simulink model "lab07q1"  (Simulink 7.1)
settings: Solver=ode45  StartTime=0.0  StopTime=100  RelTol=1e-3
InitFcn:
  | RC = 2;
  | K= 1;
  | 
  | 
  | A = [(-1/RC)*(2-K) (1/RC)*K (-1/RC);(1/RC)*K (1/RC)*K (-1/RC);(1/(2*RC))*(1+2*K) (1/(2*RC))*(1+2*K) (-1/RC)]
  | 
  | B = [(1/RC)*(2-K);(-1/RC)*K;(-1/RC)*K]
  | 
  | C = [-(1+K) -(1+K) 0;1 0 0;0 1 0;0 0 1]
  | 
  | D = [(1+K);0;0;0]
libraries: simulink x3
settings Model: Creator=ALUNO  LastModifiedBy=ALUNO

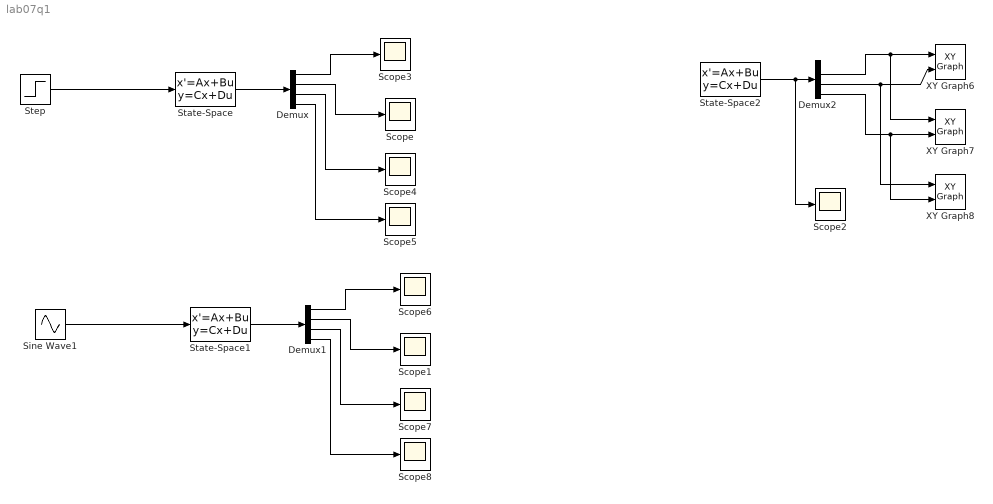
== system lab07q1 ==
  Demux : Demux
  Demux1 : Demux
  Demux2 : Demux
  Scope{,1..8} (9 alike) : Scope
      Scope2 settings: SaveName=ScopeData2
      Scope3 settings: SaveName=ScopeData3
      Scope4 settings: SaveName=ScopeData4
      Scope5 settings: SaveName=ScopeData5
      Scope6 settings: SaveName=ScopeData6
      Scope7 settings: SaveName=ScopeData7
      Scope8 settings: SaveName=ScopeData8
  Sine Wave1 : Sin  Frequency=5  SampleTime=0
  State-Space : StateSpace  A=A  B=B  C=C  D=D
  State-Space1 : StateSpace  A=A  B=B  C=C  D=D
  State-Space2 : StateSpace  A=A  B=B  C=C  D=D  X0=[4;-3;8]
  Step : Step  Time=0  SampleTime=0
  XY Graph6 : simulink/Sinks/XY Graph  SystemSampleTime=-1  xmin=-5  xmax=5  ymin=-5  ymax=5  st=-1
  XY Graph7 : simulink/Sinks/XY Graph  SystemSampleTime=-1  xmin=-5  xmax=5  ymin=-5  ymax=5  st=-1
  XY Graph8 : simulink/Sinks/XY Graph  SystemSampleTime=-1  xmin=-5  xmax=5  ymin=-5  ymax=5  st=-1
  wires:
  State-Space/1 -> Demux/1
  State-Space1/1 -> Demux1/1
  Sine Wave1/1 -> State-Space1/1
  State-Space2/1 -> Demux2/1, Scope2/1
  Demux2/2 -> XY Graph6/1, XY Graph7/1
  Demux2/3 -> XY Graph6/2, XY Graph8/1
  Demux2/4 -> XY Graph7/2, XY Graph8/2
  Step/1 -> State-Space/1
  Demux/1 -> Scope3/1
  Demux/2 -> Scope/1
  Demux/3 -> Scope4/1
  Demux/4 -> Scope5/1
  Demux1/1 -> Scope6/1
  Demux1/2 -> Scope1/1
  Demux1/3 -> Scope7/1
  Demux1/4 -> Scope8/1
